simulink model "serialTest"  (R2018a)
settings: Solver=VariableStepAuto  StartTime=0.0  StopTime=inf  RelTol=1e-3
settings Model: Creator=hal  LastModifiedBy=hal

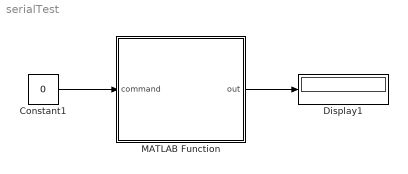
== system serialTest ==
  Constant1 : Constant  Value=0  OutDataTypeStr=double  SampleTime=0.05
  Display1 : Display
      settings: Format=decimal (Stored Integer)
  MATLAB Function : MATLAB Function  TreatAsAtomicUnit=on
  wires:
  MATLAB Function/1(out) -> Display1/1
  Constant1/1 -> MATLAB Function/1(command)

== matlab function serialTest/MATLAB Function ==
  data: out output; command input
function out = serialpassthrough(command)
    out = nan;
    coder.extrinsic('serial', 'instrfind', 'fscanf', 'num2str')
    port_arduino_motors = '/dev/ttyACM0';
    persistent COM_arduino_motors

    if isempty(COM_arduino_motors)
        if isempty(instrfind('Port', '/dev/ttyACM0'))
    %         if ~isempty(COM_arduino_motors)
    %             fclose(COM_arduino_motors);
    %             delete(COM_arduino_motors) 
    %         end
            COM_arduino_motors = serial(port_arduino_motors);
            set(COM_arduino_motors, 'Timeout', 10)
            set(COM_arduino_motors, 'BaudRate', 115200)
            set(COM_arduino_motors, 'OutputBufferSize', 1)
            set(COM_arduino_motors, 'InputBufferSize', 4)
            set(COM_arduino_motors, 'Terminator', {'CR/LF', ''});
            fclose(COM_arduino_motors);
            fopen(COM_arduino_motors);  
        else
            COM_arduino_motors = instrfind('Port', '/dev/ttyACM0');
            set(COM_arduino_motors, 'Timeout', 10)
            set(COM_arduino_motors, 'BaudRate', 115200)
            set(COM_arduino_motors, 'OutputBufferSize', 1)
            set(COM_arduino_motors, 'InputBufferSize', 4)
            set(COM_arduino_motors, 'Terminator', {'CR/LF', ''});
            fclose(COM_arduino_motors);
            fopen(COM_arduino_motors); 
        end
    end
    
    fprintf(COM_arduino_motors, num2str(command));
    temp = fscanf(COM_arduino_motors);
    out = str2double(temp);

end
